simulink model "semiactivesimulation"  (R2025b)
settings: Solver=ode4  StartTime=0.0  StopTime=5  FixedStep=0.001  RelTol=1e-3
undefined symbols (not defined in the file): k_suspension, k_tire, m_sprung, m_unsprung
settings Model: Creator=aedan  LastModifiedBy=aedan

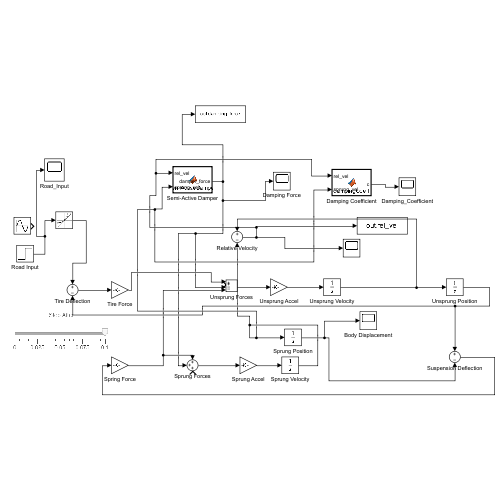
[thumbnail: Simulink's stored preview of the top-level diagram]
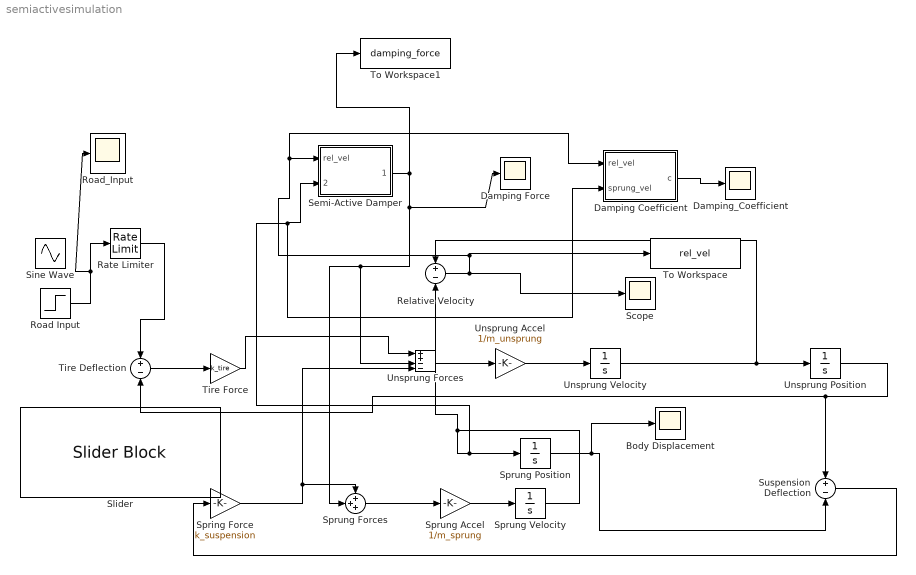
== system semiactivesimulation ==
  Body Displacement : Scope
      settings: ActiveDisplayYMinimum=-0.015964015230026583  ActiveDisplayYMaximum=0.14367613707023927
  Damping Coefficient : MATLAB Function  TreatAsAtomicUnit=on
  Damping Force : Scope
      settings: ActiveDisplayYMinimum=-525.04836391077072  ActiveDisplayYMaximum=652.87188829018066  DataLoggingVariableName=ScopeData2
  Damping_Coefficient : Scope
      settings: ActiveDisplayYMinimum=587.50000013637873  ActiveDisplayYMaximum=2712.4999988465361  DataLoggingVariableName=ScopeData3
  Rate Limiter : RateLimiter  RisingSlewLimit=0.2  FallingSlewLimit=-0.2  SampleTimeMode=inherited
  Relative Velocity : Sum  Inputs=+-
  Road Input : Step  Time=0.5  After=0.1  SampleTime=0
  Road_Input : Scope
      settings: ActiveDisplayYMinimum=-1  ActiveDisplayYMaximum=1
  Scope : Scope
      settings: ActiveDisplayYMinimum=-1  ActiveDisplayYMaximum=1  DataLoggingVariableName=ScopeData4
  Semi-Active Damper : MATLAB Function  TreatAsAtomicUnit=on
  Sine Wave : Sin  Amplitude=0.02  Frequency=4*pi  SampleTime=0
  Slider : SliderBlock  ScaleMax=0.1
  Spring Force : Gain  Gain=k_suspension
  Sprung Accel : Gain  Gain=1/m_sprung
  Sprung Forces : Sum  Inputs=+++
  Sprung Position : Integrator
  Sprung Velocity : Integrator
  Suspension Deflection : Sum  Inputs=+-
  Tire Deflection : Sum  Inputs=+-
  Tire Force : Gain  Gain=k_tire
  To Workspace : ToWorkspace  VariableName=rel_vel  SampleTime=-1
  To Workspace1 : ToWorkspace  VariableName=damping_force  SampleTime=-1
  Unsprung Accel : Gain  Gain=1/m_unsprung
  Unsprung Forces : Sum  Inputs=++--
  Unsprung Position : Integrator
  Unsprung Velocity : Integrator
  wires:
  Unsprung Velocity/1 -> Relative Velocity/1, Unsprung Position/1
  Unsprung Forces/1 -> Unsprung Accel/1
  Unsprung Accel/1 -> Unsprung Velocity/1
  Tire Force/1 -> Unsprung Forces/1
  Unsprung Position/1 -> Suspension Deflection/1, Tire Deflection/2
  Tire Deflection/1 -> Tire Force/1
  Sprung Forces/1 -> Sprung Accel/1
  Sprung Accel/1 -> Sprung Velocity/1
  Sprung Velocity/1 -> Damping Coefficient/2(sprung_vel), Semi-Active Damper/2(sprung_vel), Sprung Position/1, Relative Velocity/2
  Sprung Position/1 -> Suspension Deflection/2, Body Displacement/1
  Suspension Deflection/1 -> Spring Force/1
  Spring Force/1 -> Unsprung Forces/4, Sprung Forces/1
  Relative Velocity/1 -> Damping Coefficient/1(rel_vel), Semi-Active Damper/1(rel_vel), To Workspace/1, Scope/1
  Semi-Active Damper/1(damper_force) -> Unsprung Forces/3, Sprung Forces/2, Damping Force/1, To Workspace1/1
  Damping Coefficient/1(c) -> Damping_Coefficient/1
  Road Input/1 -> Road_Input/1, Rate Limiter/1
  Rate Limiter/1 -> Tire Deflection/1

== matlab function semiactivesimulation/Semi-Active Damper ==
  data: rel_vel input; damper_force output; sprung_vel input
function damper_force = semiActiveDamper(rel_vel, sprung_vel)
    % Proportional semi-active damping for off-road racing
    % Hard on compression (impacts), soft on extension (terrain following)
    
    damper_force = 0;  % Initialize output
    
    c_soft = 800;    % N*s/m - Extension (lets wheel drop to follow terrain)
    c_hard = 2500;   % N*s/m - Compression (controls impacts, prevents bottoming)
    
    % Blend based on compression velocity
    % Positive rel_vel = compression (wheel moving up) -> use hard damping
    % Negative rel_vel = extension (wheel dropping) -> use soft damping
    
    scale = 0.05;  % Transition smoothness (adjust as needed)
    compression_factor = tanh(rel_vel / scale);  % -1 (extension) to +1 (compression)
    
    % Map to 0-1: 0 = full extension (soft), 1 = full compression (hard)
    normalized = (compression_factor + 1) / 2;
    
    % Interpolate damping coefficient
    c = c_soft + (c_hard - c_soft) * normalized;
    
    damper_force = c * rel_vel;
end

== matlab function semiactivesimulation/Damping Coefficient ==
  data: rel_vel input; c output; sprung_vel input
function c = dampingCoeff(rel_vel, sprung_vel)
    c_soft = 800;
    c_hard = 2500;
    effectiveness = rel_vel * sprung_vel;
    scale = 0.1;
    blend_factor = tanh(effectiveness / scale);
    normalized = (blend_factor + 1) / 2;
    c = c_soft + (c_hard - c_soft) * normalized;
end
